simulink model "test_layerwall_static"  (R2018b)
settings: Solver=ode45  StartTime=0.0  StopTime=2*24*3600  RelTol=1e-3  EnableMultiTasking=on
libraries: carnot x5
settings Model: Creator=drhf  LastModifiedBy=drhf
settings DataIOCC: LimitDataPoints=on  SaveFormat=Array
settings OptimizationCC: DefaultParameterBehavior=Inlined  LifeSpan=inf
settings DebuggingCC: UnderspecifiedInitializationDetection=Classic  MergeDetectMultiDrivingBlocksExec=none  SolverPrmCheckMsg=warning  SFUnexpectedBacktrackingDiag=warning  SFNoUnconditionalDefaultTransitionDiag=warning  SFExecutionAtInitializationDiag=none
settings HardwareCC: ProdBitPerPointer=32  ProdBitPerSizeT=32  ProdBitPerPtrDiffT=32  ProdLargestAtomicFloat=None  ProdIntDivRoundTo=Undefined  ProdEndianess=Unspecified  ProdWordSize=32  ProdHWDeviceType=32-bit Generic
settings ModelReferenceCC: PropagateSignalLabelsOutOfModel=off
settings SFSimCC: SimUseLocalCustomCode=off
settings RTWCC: RTWUseLocalCustomCode=off
settings CodeAppCC: StateflowObjectComments=on
settings GRTTargetCC: TargetLangStandard=C89/C90 (ANSI)  GeneratePreprocessorConditionals=Disable all
settings ConfigComp: CovMetricSettings=dw  CovHtmlReporting=on  CovSaveCumulativeToWorkspaceVar=on  CovSaveSingleToWorkspaceVar=on  CovExternalEMLEnable=off

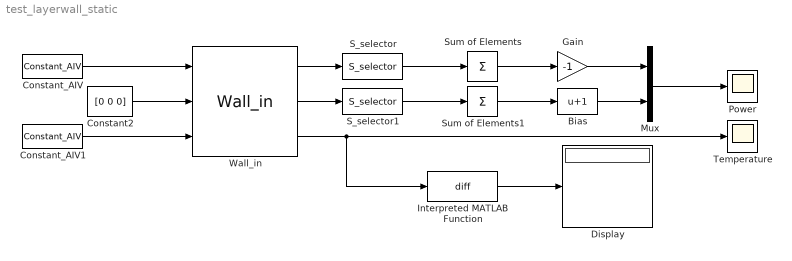
== system test_layerwall_static ==
  Bias : Bias  Bias=1
  Constant2 : Constant  Value=[0 0 0]
  Constant_AIV : carnot/Source/Ventilation/Constant_AIV  Tsens=20  Tcon=20  Trad=20  mw=0.012  mco=0.01  rhoair=1.2  cpair=1004  pair=100000  nair=0.5
      settings: SourceProductName=Carnot
  Constant_AIV1 : carnot/Source/Ventilation/Constant_AIV  Tsens=0  Tcon=0  Trad=0  mw=0.012  mco=0.01  rhoair=1.2  cpair=1004  pair=100000  nair=0.5
      settings: SourceProductName=Carnot
  Display : Display
  Gain : Gain  Gain=-1
  Interpreted MATLAB Function : MATLABFcn  MATLABFcn=diff
  Mux : Mux  Inputs=2
  Power : Scope
  S_selector : carnot/Outputs/S_selector  e1=off  e2=off  e3=off  e4=off  e5=off  e6=off  e7=on  e8=on  e9=off  e10=off  e11=off  e12=off  e13=off
      settings: SourceProductName=Carnot
  S_selector1 : carnot/Outputs/S_selector  e1=off  e2=off  e3=off  e4=off  e5=off  e6=off  e7=on  e8=on  e9=off  e10=off  e11=off  e12=off  e13=off
      settings: SourceProductName=Carnot
  Sum of Elements : Sum  Inputs=+
  Sum of Elements1 : Sum  Inputs=+
  Temperature : Scope
  Wall_in : carnot/Basic/Thermal_Models/Wall_in  wallsize=[10 10]  d=[0.1 0.1 0.1]  cond=[1 1 1]  cwall=[0.28 0.28 0.28]*3600  rho=[2000 200 2000]  emission_in=.96  dactive=[0.075 0.15 0.225]  t0=10  tau=10*3600
      settings: SourceProductName=Carnot
  wires:
  Constant2/1 -> Wall_in/2
  Wall_in/1 -> S_selector/1
  Wall_in/2 -> S_selector1/1
  Mux/1 -> Power/1
  Constant_AIV/1 -> Wall_in/1
  Constant_AIV1/1 -> Wall_in/3
  S_selector/1 -> Sum of Elements/1
  S_selector1/1 -> Sum of Elements1/1
  Sum of Elements/1 -> Gain/1
  Sum of Elements1/1 -> Bias/1
  Wall_in/3 -> Interpreted MATLAB Function/1, Temperature/1
  Bias/1 -> Mux/2
  Gain/1 -> Mux/1
  Interpreted MATLAB Function/1 -> Display/1
